simulink library "INT_MRly_VD"  (R2016b)
settings: Solver=VariableStepAuto  StartTime=0.0  StopTime=10.0  RelTol=1e-3
settings Model: Creator=Administrator  LastModifiedBy=Administrator

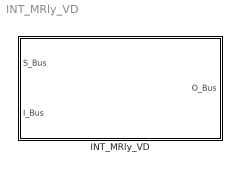
== system INT_MRly_VD ==
  INT_MRly_VD : Subsystem

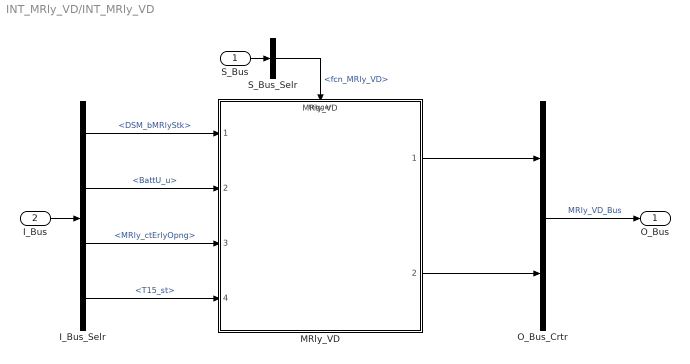
== system INT_MRly_VD/INT_MRly_VD ==
  S_Bus : Inport
  I_Bus : Inport  Port=2
  I_Bus_Selr : BusSelector  OutputSignals=DSM_bMRlyStk,BattU_u,MRly_ctErlyOpng,T15_st
  MRly_VD : ModelReference  ModelNameDialog=MRly_VD  SimulationMode=Normal  ModelReferenceVersion=1.12  TriggerPortName=function  TriggerPortTriggerType=function-call  TriggerPortStatesWhenEnabling=held
  O_Bus_Crtr : BusCreator  Inputs=2
  S_Bus_Selr : BusSelector  OutputSignals=fcn_MRly_VD
  O_Bus : Outport
  wires:
  S_Bus_Selr/1 -> MRly_VD/Trigger  "<fcn_MRly_VD>"
  S_Bus/1 -> S_Bus_Selr/1
  I_Bus/1 -> I_Bus_Selr/1
  I_Bus_Selr/1 -> MRly_VD/1  "<DSM_bMRlyStk>"
  I_Bus_Selr/2 -> MRly_VD/2  "<BattU_u>"
  I_Bus_Selr/3 -> MRly_VD/3  "<MRly_ctErlyOpng>"
  I_Bus_Selr/4 -> MRly_VD/4  "<T15_st>"
  O_Bus_Crtr/1 -> O_Bus/1  "MRly_VD_Bus"
  MRly_VD/1 -> O_Bus_Crtr/1
  MRly_VD/2 -> O_Bus_Crtr/2
